simulink model "coolingskid_digitaltwin3"  (R2026a)
settings: Solver=VariableStepAuto  StopTime=10000
libraries: fl_lib x33, SimscapeFluids_lib x13, nesl_utility x12, slpidlib x1
settings Model: Creator=novik  LastModifiedBy=novik
settings SolverCC: MaxConsecutiveMinStep=2

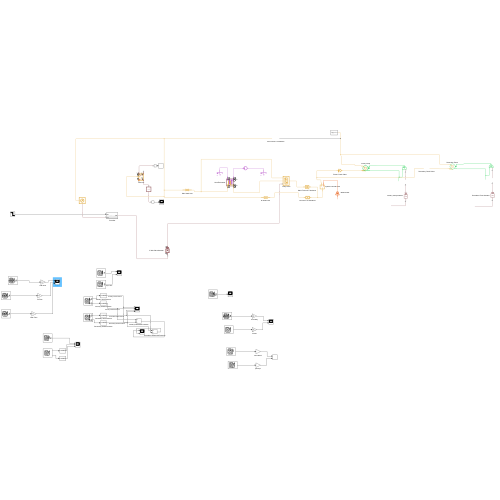
[thumbnail: Simulink's stored preview of the top-level diagram]
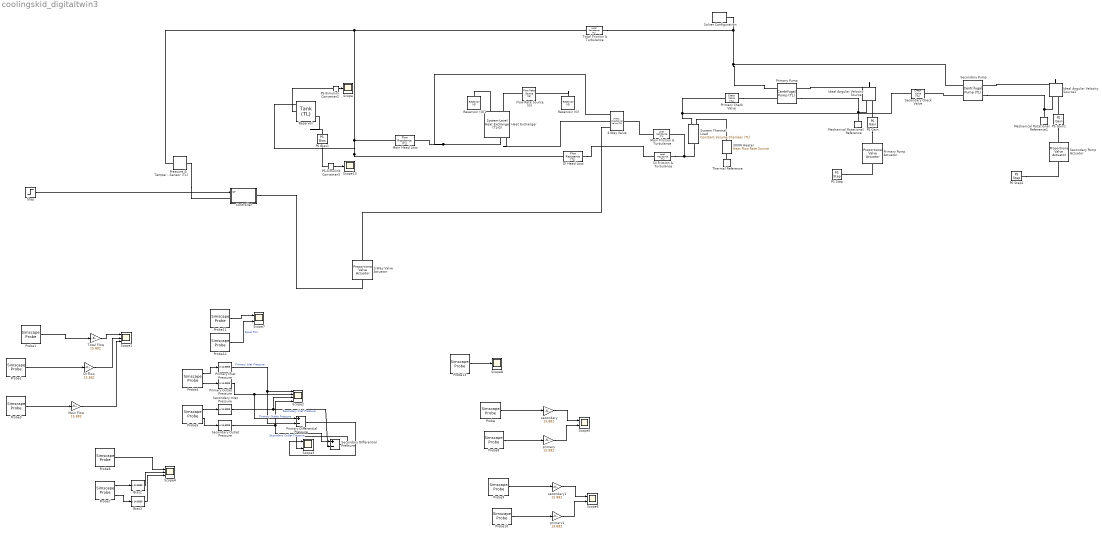
== system coolingskid_digitaltwin3 ==
  3-Way Valve : SimscapeFluids_lib/Thermal Liquid/Valves & Orifices/Directional Control Valves/3-Way Directional Valve (TL)  open_orifices_pos=fluids.thermal_liquid.valves.directional_control_valves.enum.OpenOrifices3Way.PA  open_orifices_neg=fluids.thermal_liquid.valves.directional_control_valves.enum.OpenOrifices3Way.AT  area_spec=fluids.thermal_liquid.valves.directional_control_valves.enum.area_spec.identical  valve_spec=fluids.thermal_liquid.valves.directional_control_valves.enum.ValveSpec.Linear  del_S_max=3e-3 m  area_max=0.502654824574 in^2  del_S_TLU=[0, .00125, .0025, .00375, .005] m  valve_area_TLU=[1e-10, 1e-05, 4e-05, 8e-05, .0001] m^2  del_S_flow_TLU=[0, .00125, .0025, .00375, .005] m  p_diff_TLU=[-.1, .3, .5, .7] MPa  vol_flow_TLU=[-9.05e-10, 1.57e-09, 2.02e-09, 2.39e-09; -9.05e-05, .000157, .000202, .000239; -.000362, .000627, .00081, .000958; -.000724, .00125, .00162, .00192; -.000905, .00156, .002, .00239] m^3/s  mdot_TLU=1e3 * [-9.05e-10, 1.57e-09, 2.02e-09, 2.39e-09; -9.05e-05, .000157, .000202, .000239; -.000362, .000627, .00081, .000958; -.000724, .00125, .00162, .00192; -.000905, .00156, .002, .00239] kg/s  T_ref_in=293.15 K  p_ref_in=0.101325 MPa  area_leak=1e-20 in^2  Cd=1  Re_c=1  smoothing_factor=0.01  pressure_recovery=false  area=0.533266503391 in^2  S_max_PA=5e-3 m  del_S_max_PA=0.005 m  area_max_PA=1e-4 m^2  del_S_TLU_PA=[0, .00125, .0025, .00375, .005] m  valve_area_TLU_PA=[1e-10, 1e-05, 4e-05, 8e-05, .0001] m^2  del_S_flow_TLU_PA=[0, .00125, .0025, .00375, .005] m  p_diff_TLU_PA=[-.1, .3, .5, .7] MPa  vol_flow_TLU_PA=[-9.05e-10, 1.57e-09, 2.02e-09, 2.39e-09; -9.05e-05, .000157, .000202, .000239; -.000362, .000627, .00081, .000958; -.000724, .00125, .00162, .00192; -.000905, .00156, .002, .00239] m^3/s  mdot_TLU_PA=1e3 * [-9.05e-10, 1.57e-09, 2.02e-09, 2.39e-09; -9.05e-05, .000157, .000202, .000239; -.000362, .000627, .00081, .000958; -.000724, .00125, .00162, .00192; -.000905, .00156, .002, .00239] kg/s  S_max_AT=0 m  del_S_max_AT=0.005 m  area_max_AT=1e-4 m^2  del_S_TLU_AT=[0, .00125, .0025, .00375, .005] m  valve_area_TLU_AT=[1e-10, 1e-05, 4e-05, 8e-05, .0001] m^2  del_S_flow_TLU_AT=[0, .00125, .0025, .00375, .005] m  p_diff_TLU_AT=[-.1, .3, .5, .7] MPa  vol_flow_TLU_AT=[-9.05e-10, 1.57e-09, 2.02e-09, 2.39e-09; -9.05e-05, .000157, .000202, .000239; -.000362, .000627, .00081, .000958; -.000724, .00125, .00162, .00192; -.000905, .00156, .002, .00239] m^3/s  mdot_TLU_AT=1e3 * [-9.05e-10, 1.57e-09, 2.02e-09, 2.39e-09; -9.05e-05, .000157, .000202, .000239; -.000362, .000627, .00081, .000958; -.000724, .00125, .00162, .00192; -.000905, .00156, .002, .00239] kg/s  S_max_PT=4.5e-3 m  del_S_max_PT=0.005 m  area_max_PT=1e-4 m^2  del_S_TLU_PT=[0, .00125, .0025, .00375, .005] m  valve_area_TLU_PT=[1e-10, 1e-05, 4e-05, 8e-05, .0001] m^2  del_S_flow_TLU_PT=[0, .00125, .0025, .00375, .005] m  p_diff_TLU_PT=[-.1, .3, .5, .7] MPa  vol_flow_TLU_PT=[-9.05e-10, 1.57e-09, 2.02e-09, 2.39e-09; -9.05e-05, .000157, .000202, .000239; -.000362, .000627, .00081, .000958; -.000724, .00125, .00162, .00192; -.000905, .00156, .002, .00239] m^3/s  mdot_TLU_PT=1e3 * [-9.05e-10, 1.57e-09, 2.02e-09, 2.39e-09; -9.05e-05, .000157, .000202, .000239; -.000362, .000627, .00081, .000958; -.000724, .00125, .00162, .00192; -.000905, .00156, .002, .00239] kg/s
  3-Way Valve Actuator : SimscapeFluids_lib/Valve Actuators/Proportional Valve Actuator  gain=5e-3 m  time_constant=3 s  valve_stroke=0.005 m
  300W Heater : fl_lib/Thermal/Thermal Sources/Heat Flow Rate Source  heat_flow=300 W
  Bias2 : Bias  Bias=-14.6959  SaturateOnIntegerOverflow=off
  Bias3 : Bias  Bias=-14.6959  SaturateOnIntegerOverflow=off
  Controller : Subsystem
  DI Flow : Gain  Gain=15.882
  DI Friction & Turbulance : SimscapeFluids_lib/Thermal Liquid/Pipes & Fittings/Local Resistance (TL)  resistance_loss_spec=fluids.thermal_liquid.pipes_fittings.enum.ResistanceLossSpec.Constant  loss_coeff_AB=0.041443  loss_coeff_BA=0.041443  Re_TLU=[-500, -200, -100, -50, -40, -30, -20, -10, 10, 20, 30, 40, 50, 100, 200, 500, 1000, 2000]  loss_coeff_TLU=[.65, .75, .9, 1.15, 1.35, 1.65, 2.3, 3.1, 4, 2.7, 1.8, 1.46, 1.3, .9, .65, .42, .3, .2]  flow_area=0.533266503391 in^2  Re_c=3380
  DI Head Loss : fl_lib/Thermal Liquid/Elements/Flow Resistance (TL)  delta_p_nominal=7.908 psi  mdot_nominal=0.05667 kg/s  area=0.533266503391 in^2  laminar_fraction=1e-3
  Flow Rate Source (G) : fl_lib/Gas/Sources/Flow Rate Source (G)  source_type=foundation.enum.constant_controlled.constant  flow_type=foundation.enum.mass_volumetric_flow.mass  mass_flow=5 kg/s  volumetric_flow=0 m^3/s  volumetric_flow_conditions=foundation.enum.volumetric_flow_conditions.standard  p_std=0.101325 MPa  T_std=20 degC  power_spec=foundation.enum.power_spec.isentropic  area_A=0.01 m^2  area_B=0.01 m^2
  Heat Exchanger : SimscapeFluids_lib/Heat Exchangers/Thermal Liquid - Gas/System-Level Heat Exchanger (TL-G)  flow_arrangement=fluids.heat_exchangers.enum.SystemLevelFlowArrangementTLG.Counter  wall_thermal_mass=false  mass_wall=1 kg  cp_wall=490 J/(K*kg)  nominal_init_wall=true  T_wall_init=293.15 K  area_A1=0.533266503391 in^2  area_B1=0.533266503391 in^2  area_A2=0.01 m^2  area_B2=0.01 m^2  operating_condition_TL=fluids.heat_exchangers.enum.SystemLevelOperatingConditionTLG.Cooling  mdot_nominal_TL=0.315450833333 kg/s  delta_p_nominal_TL=2.08 psi  p_in_nominal_TL=23.5 psi  T_in_nominal_TL=43.54 degC  capacity_spec_TL=fluids.heat_exchangers.enum.SystemLevelCapacitySpec.OutletCondition  Q_nominal=1 kW  T_out_nominal_TL=26.87 degC  volume_TL=.25 gal  nominal_init_TL=false  p_init_TL=1 atm  T_init_TL=25 degC  mdot_nominal_G=5 kg/s  delta_p_nominal_G=0.001 MPa  p_in_nominal_G=0.101325 MPa  T_in_nominal_G=25 degC  volume_G=0.1 m^3  nominal_init_G=true  p_init_G=0.101325 MPa  T_init_G=293.15 K  a_TL=0.023  b_TL=0.8  c_TL=0.33  a_G=0.023  b_G=0.8  c_G=0.33
  Ideal Angular Velocity Source : fl_lib/Mechanical/Mechanical Sources/Ideal Angular Velocity Source
  Ideal Angular Velocity Source1 : fl_lib/Mechanical/Mechanical Sources/Ideal Angular Velocity Source
  Main Flow : Gain  Gain=15.882
  Main Friction & Turbulance : SimscapeFluids_lib/Thermal Liquid/Pipes & Fittings/Local Resistance (TL)  resistance_loss_spec=fluids.thermal_liquid.pipes_fittings.enum.ResistanceLossSpec.Constant  loss_coeff_AB=0.026994  loss_coeff_BA=0.026994  Re_TLU=[-500, -200, -100, -50, -40, -30, -20, -10, 10, 20, 30, 40, 50, 100, 200, 500, 1000, 2000]  loss_coeff_TLU=[.65, .75, .9, 1.15, 1.35, 1.65, 2.3, 3.1, 4, 2.7, 1.8, 1.46, 1.3, .9, .65, .42, .3, .2]  flow_area=0.533266503391 in^2  Re_c=18778
  Main Head Loss : fl_lib/Thermal Liquid/Elements/Flow Resistance (TL)  delta_p_nominal=5.94 psi  mdot_nominal=0.315450833333 kg/s  area=0.533266503391 in^2  laminar_fraction=1e-3
  Mechanical Rotational Reference : fl_lib/Mechanical/Rotational Elements/Mechanical Rotational Reference
  Mechanical Rotational Reference1 : fl_lib/Mechanical/Rotational Elements/Mechanical Rotational Reference
  PS Bias1 : fl_lib/Physical Signals/Functions/PS Bias  bias=-273.15 K
  PS Gain : fl_lib/Physical Signals/Functions/PS Gain  gain=1 1/(m*s)
  PS Gain1 : fl_lib/Physical Signals/Functions/PS Gain  gain=1 1/(m*s)
  PS Step : fl_lib/Physical Signals/Sources/PS Step  step_time=5000 s  initial_value=1  final_value=0
  PS Step1 : fl_lib/Physical Signals/Sources/PS Step  step_time=5000 s  initial_value=0  final_value=1
  PS-Simulink Converter2 : nesl_utility/PS-Simulink Converter  PhysicalDomain=network_engine_domain  SubClassName=ps_output  LeftPortType=input  RightPortType=output  PseudoPeriodic=off  Frequencies=[]  VectorFormat=inherit  Unit=inherit  AffineConversion=off
  PS-Simulink Converter3 : nesl_utility/PS-Simulink Converter  PhysicalDomain=network_engine_domain  SubClassName=ps_output  LeftPortType=input  RightPortType=output  PseudoPeriodic=off  Frequencies=[]  VectorFormat=inherit  Unit=inherit  AffineConversion=off
  Pressure & Temperature Sensor (TL) : fl_lib/Thermal Liquid/Sensors/Pressure & Temperature Sensor (TL)  reference=foundation.enum.MeasurementReference.absolute  pressure=false  pressure_spec=foundation.enum.PressureMeasementSpec.Absolute  temperature=true
  Primary Check Valve : SimscapeFluids_lib/Thermal Liquid/Valves & Orifices/Directional Control Valves/Check Valve (TL)  opening_spec=fluids.thermal_liquid.valves.enum.PressureOpeningSpec.Linear  pressure_spec=fluids.thermal_liquid.valves.enum.PressureControlSpec.PressureDifferential  p_crack_gauge=0.1 MPa  p_crack_differential=0.01 psi  press_max_gauge=0.2 MPa  press_max_differential=0.21 psi  area_max=0.5 in^2  area_leak=1e-10 m^2  p_diff_TLU=[0.01 : 0.01 : 0.1] MPa  valve_area_TLU=[1e-10, 1e-05, 2e-05, 3e-05, 4e-05, 5e-05, 6e-05, 7.5e-05, 8.5e-05, .0001] m^2  vol_flow_TLU=[.000358, .045, .11, .191, .284, .39, .505, .63, .764, .905] .* 1e-3 m^3/s  area=0.533266503391 in^2  Cd=1  Re_c=1  smoothing_factor=0.01  pressure_recovery=false  opening_dynamics=false  tau=0.1 s
  Primary Differential Pressure : Sum  Inputs=+-
  Primary Inlet Pressure : Bias  Bias=-14.6959  SaturateOnIntegerOverflow=off
  Primary Outlet Pressure : Bias  Bias=-14.6959  SaturateOnIntegerOverflow=off
  Primary Pump : SimscapeFluids_lib/Thermal Liquid/Pumps & Motors/Centrifugal Pump (TL)  pump_parameterization=fluids.thermal_liquid.pumps_motors.enum.CentrifugalPumpParameterization.Nominal  capacity_ref_nominal=5.9 gpm  head_ref_nominal=19 ft  power_ref_nominal=0.02811289 kW  head_ref_max=20.7652445345097 ft  capacity_ref_max=31 gpm  omega_ref_analytic=1770 rpm  flow_rate_1D_TLU=[16.67, 30, 40, 53.33, 66.67, 83.33] lpm  head_1D_TLU=[50, 47.5, 45, 40, 35, 25] m  power_1D_TLU=[.6, .75, .85, .93, .98, .99] kW  omega_ref_1D=3500 rpm  rho_ref_1D=998.21 kg/m^3  omega_threshold_factor=1e-2  flow_rate_2D_TLU=[16.67, 23.33, 30, 40, 53.33, 60] lpm  omega_2D_TLU=[2450, 2800, 3150, 3500] rpm  head_2D_TLU=[25, 32.7, 42.5, 50; 24, 31.7, 41, 49; 22.7, 30.5, 39, 47.5; 20, 28, 36, 45; 15.7, 24, 32, 40; 12.5, 21, 29.5, 37.5] m  power_2D_TLU=[.28, .38, .5, .6; .31, .41, .55, .68; .33, .44, .6, .75; .36, .48, .65, .83; .38, .53, .72, .93; .39, .55, .75, .97] kW  rho_ref_2D=998.21 kg/m^3  diameter_ratio=1  mech_orientation=fluids.thermal_liquid.pumps_motors.enum.CentrifugalPumpMechOrientation.Positive  area=0.533266503391 in^2  operation_check=simscape.enum.assert.action.none
  Primary Pump Actuator : SimscapeFluids_lib/Valve Actuators/Proportional Valve Actuator  gain=185.3539665617978 m  time_constant=8 s  valve_stroke=185.3539665617978 m
  Probe : SimscapeProbe  BoundBlock=69  Variables="{\"mdot_A\":{\"Probing\":\"ON\"}}"
  Probe1 : SimscapeProbe  BoundBlock=421  Variables="{\"mdot_A\":{\"Probing\":\"ON\"}}"
  Probe10 : SimscapeProbe  BoundBlock=219  Variables="{\"O\":{\"Probing\":\"ON\"}}"
  Probe11 : SimscapeProbe  BoundBlock=406  Variables="{\"A.T\":{\"Unit\":\"degC\",\"Probing\":\"ON\"}}"
  Probe12 : SimscapeProbe  BoundBlock=118  Variables="{\"S\":{\"Probing\":\"ON\"}}"
  Probe13 : SimscapeProbe  BoundBlock=77  Variables="{\"B.p\":{\"Unit\":\"psi\",\"Probing\":\"ON\"}}"
  Probe2 : SimscapeProbe  BoundBlock=77  Variables="{\"mdot_A\":{\"Probing\":\"ON\"}}"
  Probe3 : SimscapeProbe  BoundBlock=73  Variables="{\"mdot_A\":{\"Probing\":\"ON\"}}"
  Probe4 : SimscapeProbe  BoundBlock=69  Variables="{\"A.p\":{\"Unit\":\"psi\",\"Probing\":\"ON\"},\"B.p\":{\"Unit\":\"psi\",\"Probing\":\"ON\"}}"
  Probe5 : SimscapeProbe  BoundBlock=236  Variables="{\"A.p\":{\"Unit\":\"psi\",\"Probing\":\"ON\"},\"B.p\":{\"Unit\":\"psi\",\"Probing\":\"ON\"},\"mdot_A\":{\"Probing\":\"OFF\"},\"mdot_B\":{\"Probing\":\"OFF\"}}"
  Probe6 : SimscapeProbe  BoundBlock=69  Variables="{\"R.w\":{\"Unit\":\"rpm\",\"Probing\":\"ON\"}}"
  Probe7 : SimscapeProbe  BoundBlock=69  Variables="{\"A.p\":{\"Unit\":\"psi\",\"Probing\":\"ON\"},\"B.p\":{\"Unit\":\"psi\",\"Probing\":\"ON\"}}"
  Probe8 : SimscapeProbe  BoundBlock=236  Variables="{\"mdot_A\":{\"Probing\":\"ON\"}}"
  Probe9 : SimscapeProbe  BoundBlock=240  Variables="{\"O\":{\"Probing\":\"ON\"}}"
  Reservoir : SimscapeFluids_lib/Thermal Liquid/Tanks & Accumulators/Tank (TL)  num_inlet=fluids.thermal_liquid.tanks_accumulators.enum.NumInlet.One  pressure_spec=fluids.thermal_liquid.tanks_accumulators.enum.TankPressureSpec.Atmospheric  tank_pressure=0.101325 MPa  volume_spec=fluids.thermal_liquid.tanks_accumulators.enum.TankVolumeSpec.Constant  tank_area=144 in^2  level_TLU=[0, 3, 5] m  volume_TLU=[0, 4, 6] m^3  inlet_height_A=0.1 in  inlet_area_A=.78 in^2  inlet_heights_AB=[.1, .1] m  inlet_areas_AB=[.01, .01] m^2  inlet_heights_ABC=[.1, .1, .1] m  inlet_areas_ABC=[.01, .01, .01] m^2  inlet_heights_ABCD=0.1 * ones(1, 4) m  inlet_areas_ABCD=0.01 * ones(1, 4) m^2  inlet_heights_ABCDE=0.1 * ones(1, 5) m  inlet_areas_ABCDE=0.01 * ones(1, 5) m^2  inlet_heights_ABCDEF=0.1 * ones(1, 6) m  inlet_areas_ABCDEF=0.01 * ones(1, 6) m^2  level_check=simscape.enum.assert.action.error  capacity_check=simscape.enum.assert.action.none  max_capacity=10 m^3  g=9.81 m/s^2  level_specify=on  level_priority=None  level=5 m  level_nominal_specify=off  level_nominal_value=1  level_nominal_unit=m  volume_specify=on  volume_priority=High  volume=4 gal  volume_nominal_specify=off  volume_nominal_value=4  volume_nominal_unit=gal  mass_specify=off  mass_priority=None  mass=5000 kg  mass_nominal_specify=off  mass_nominal_value=1  mass_nominal_unit=kg  T_I_specify=on  T_I_priority=High  T_I=25 degC  T_I_nominal_specify=off  T_I_nominal_value=1  T_I_nominal_unit=K
  Reservoir (G) : fl_lib/Gas/Elements/Reservoir (G)  pressure_input=false  pressure_spec=foundation.enum.pressure_spec.atmospheric  reservoir_pressure=0.101325 MPa  temperature_input=false  reservoir_temperature=25 degC  area_A=0.01 m^2  input_error_spec=foundation.enum.input_range_error.warn
  Reservoir (G)1 : fl_lib/Gas/Elements/Reservoir (G)  pressure_input=false  pressure_spec=foundation.enum.pressure_spec.atmospheric  reservoir_pressure=0.101325 MPa  temperature_input=false  reservoir_temperature=293.15 degC  area_A=0.01 m^2  input_error_spec=foundation.enum.input_range_error.warn
  Scope : Scope
      settings: ActiveDisplayYMinimum=0.01508889434891056  ActiveDisplayYMaximum=0.015292483650747727  DataLoggingVariableName=ScopeData5
  Scope1 : Scope  NumInputPorts=3
      settings: Title=Total Flow  ActiveDisplayYMinimum=6.1667689576391185  ActiveDisplayYMaximum=6.8690776559533306  YLabel=Flow (GPM)
  Scope13 : Scope
      settings: ActiveDisplayYMinimum=25.00428838938462  ActiveDisplayYMaximum=25.152201193488068  DataLoggingVariableName=ScopeData10
  Scope2 : Scope  NumInputPorts=4
      settings: ActiveDisplayYMinimum=-0.7997937937117674  ActiveDisplayYMaximum=9.44542911175904  YLabel=Pressure (psi)  DataLoggingVariableName=Pressure_Pump_PortA  DataLoggingSaveFormat=Array
  Scope{3,5..7} (4 alike) : Scope  NumInputPorts=2
      Scope3 settings: Title=Primary Differential Pressure  ActiveDisplayYMinimum=-1.0243925853144504  ActiveDisplayYMaximum=9.2217499271304018  YLabel=Pressure (psi)  DataLoggingVariableName=Pressure_Pump_PortA1  DataLoggingSaveFormat=Array
      Scope5 settings: ActiveDisplayYMinimum=1.077490568227446  ActiveDisplayYMaximum=7.5374604811752661  DataLoggingVariableName=ScopeData2
      Scope6 settings: ActiveDisplayYMinimum=-367.97396371923259  ActiveDisplayYMaximum=3311.7656592293288  DataLoggingVariableName=ScopeData3
      Scope7 settings: Title=Temperature  ActiveDisplayYMinimum=21.124726674032793  ActiveDisplayYMaximum=47.999112623350065  YLabel=Temp °C
  Scope4 : Scope  NumInputPorts=3
      settings: ActiveDisplayString=3  Title=Pump Outlet Pressure  ActiveDisplayYMinimum=-5.5996179237023327  ActiveDisplayYMaximum=310.42338582580572  YLabel=Pressure (psi)  DataLoggingVariableName=Pressure_Pump_PortA2  DataLoggingSaveFormat=Array
  Scope8 : Scope
      settings: ActiveDisplayYMinimum=14.00401391479239  ActiveDisplayYMaximum=15.025108344851473  YLabel=Flow (GPM)  DataLoggingVariableName=ScopeData4
  Secondary Check Valve : SimscapeFluids_lib/Thermal Liquid/Valves & Orifices/Directional Control Valves/Check Valve (TL)  opening_spec=fluids.thermal_liquid.valves.enum.PressureOpeningSpec.Linear  pressure_spec=fluids.thermal_liquid.valves.enum.PressureControlSpec.PressureDifferential  p_crack_gauge=0.1 MPa  p_crack_differential=0.01 psi  press_max_gauge=0.2 MPa  press_max_differential=0.21 psi  area_max=0.5 in^2  area_leak=1e-10 m^2  p_diff_TLU=[0.01 : 0.01 : 0.1] MPa  valve_area_TLU=[1e-10, 1e-05, 2e-05, 3e-05, 4e-05, 5e-05, 6e-05, 7.5e-05, 8.5e-05, .0001] m^2  vol_flow_TLU=[.000358, .045, .11, .191, .284, .39, .505, .63, .764, .905] .* 1e-3 m^3/s  area=0.533266503391 in^2  Cd=1  Re_c=1  smoothing_factor=0.01  pressure_recovery=false  opening_dynamics=false  tau=0.1 s
  Secondary Differential Pressure : Sum  Inputs=+-
  Secondary Inlet Pressure : Bias  Bias=-14.6959  SaturateOnIntegerOverflow=off
  Secondary Outlet Pressure : Bias  Bias=-14.6959  SaturateOnIntegerOverflow=off
  Secondary Pump : SimscapeFluids_lib/Thermal Liquid/Pumps & Motors/Centrifugal Pump (TL)  pump_parameterization=fluids.thermal_liquid.pumps_motors.enum.CentrifugalPumpParameterization.Nominal  capacity_ref_nominal=5.9 gpm  head_ref_nominal=19 ft  power_ref_nominal=0.02811289 kW  head_ref_max=20.7652445345097 ft  capacity_ref_max=31 gpm  omega_ref_analytic=1770 rpm  flow_rate_1D_TLU=[16.67, 30, 40, 53.33, 66.67, 83.33] lpm  head_1D_TLU=[50, 47.5, 45, 40, 35, 25] m  power_1D_TLU=[.6, .75, .85, .93, .98, .99] kW  omega_ref_1D=3500 rpm  rho_ref_1D=998.21 kg/m^3  omega_threshold_factor=1e-2  flow_rate_2D_TLU=[16.67, 23.33, 30, 40, 53.33, 60] lpm  omega_2D_TLU=[2450, 2800, 3150, 3500] rpm  head_2D_TLU=[25, 32.7, 42.5, 50; 24, 31.7, 41, 49; 22.7, 30.5, 39, 47.5; 20, 28, 36, 45; 15.7, 24, 32, 40; 12.5, 21, 29.5, 37.5] m  power_2D_TLU=[.28, .38, .5, .6; .31, .41, .55, .68; .33, .44, .6, .75; .36, .48, .65, .83; .38, .53, .72, .93; .39, .55, .75, .97] kW  rho_ref_2D=998.21 kg/m^3  diameter_ratio=1  mech_orientation=fluids.thermal_liquid.pumps_motors.enum.CentrifugalPumpMechOrientation.Positive  area=0.533266503391 in^2  operation_check=simscape.enum.assert.action.none
  Secondary Pump Actuator : SimscapeFluids_lib/Valve Actuators/Proportional Valve Actuator  gain=185.3539665617978 m  time_constant=8 s  valve_stroke=185.3539665617978 m
  Solver Configuration : nesl_utility/Solver Configuration  PhysicalDomain=network_engine_domain  SubClassName=solver  LeftPortType=input  RightPortType=generic  Tones=[]  Harmonics=[]  SimulateNoise=off  Profile=off  UseLocalSampling=off  EnableSwitchedLinearOptims=on  FrequencyDomain=off  UseCCode=off  RelTol=0.001  AbsTol=0.001  MinStep=1e-09  ToWorkspace=off  RevertToSquareIcSolve=off  NumHomotopyIterations=100  PhasorMode=off  PhasorModeNumHarmonics=1  ConsistencySolver=NEWTON_XTOL_AFTER_FTOL  CanonicalOrdering=CANONICAL  OptimizeIntermediates=OPTIMIZED  IndexReductionMethod=DerivativeReplacement  DoDC=off  ResidualTolerance=1e-09  ConsistencyTolSource=GLOBAL  ConsistencyAbsTol=0.001  ConsistencyRelTol=0.001  ConsistencyTolFactor=0.001  UseLocalSolver=off  LocalSolverChoice=NE_TRAPEZOIDAL_ADVANCER  ResolveIndetEquations=on  FunctionEvalNumThread=1  LocalSolverSampleTime=0.001  DoFixedCost=off  MaxNonlinIter=3  MaxModeIter=2  ComputeImpulses=off  ImpulseIterations=2  LinearAlgebra=auto  LinearAlgebraNumThread=0  EquationFormulation=NE_TIME_EF  DelaysMemoryBudget=1024  AutomaticFiltering=on  FilteringTimeConstant=0.001  PartitionStorageMethod=AS_NEEDED  PartitionMemoryBudget=1024  PartitionMethod=FAST  MultibodyUseLocalSolver=off  MultibodyLocalSolverChoice=ODE1  MultibodyLocalSolverSampleTime=0.001
  Step : Step  Time=6000  InitialValue=45  FinalValue=37  SampleTime=0
  System Thermal Load : fl_lib/Thermal Liquid/Elements/Constant Volume Chamber (TL)  volume=4.38 gal  num_ports=foundation.enum.num_ports.two  area_A=0.533266503391 in^2  area_B=0.533266503391 in^2  area_C=0.01 m^2  area_D=0.01 m^2  p_I_specify=off  p_I_priority=High  p_I=0.101325 MPa  p_I_nominal_specify=off  p_I_nominal_value=1  p_I_nominal_unit=MPa  T_I_specify=off  T_I_priority=High  T_I=293.15 K  T_I_nominal_specify=off  T_I_nominal_value=1  T_I_nominal_unit=K  u_I_specify=off  u_I_priority=None  u_I=83.906 kJ/kg  u_I_nominal_specify=off  u_I_nominal_value=1  u_I_nominal_unit=kJ/kg  rho_I_specify=off  rho_I_priority=None  rho_I=998.21 kg/m^3  rho_I_nominal_specify=off  rho_I_nominal_value=1  rho_I_nominal_unit=kg/m^3
  Thermal Reference : fl_lib/Thermal/Thermal Elements/Thermal Reference
  "Total Flow " : Gain  Gain=15.882
  Total Friction & Turbulance : SimscapeFluids_lib/Thermal Liquid/Pipes & Fittings/Local Resistance (TL)  resistance_loss_spec=fluids.thermal_liquid.pipes_fittings.enum.ResistanceLossSpec.Constant  loss_coeff_AB=0.025900  loss_coeff_BA=0.025900  Re_TLU=[-500, -200, -100, -50, -40, -30, -20, -10, 10, 20, 30, 40, 50, 100, 200, 500, 1000, 2000]  loss_coeff_TLU=[.65, .75, .9, 1.15, 1.35, 1.65, 2.3, 3.1, 4, 2.7, 1.8, 1.46, 1.3, .9, .65, .42, .3, .2]  flow_area=0.533266503391 in^2  Re_c=22159
  primary : Gain  Gain=15.882
  primary1 : Gain  Gain=15.882
  secondary : Gain  Gain=15.882
  secondary1 : Gain  Gain=15.882
  wires:
  "Total Flow "/1 -> Scope1/1
  Probe2/1 -> DI Flow/1
  DI Flow/1 -> Scope1/2
  Probe3/1 -> Main Flow/1
  Main Flow/1 -> Scope1/3
  Probe5/1 -> Secondary Inlet Pressure/1
  Secondary Inlet Pressure/1 -> Secondary Differential Pressure/2, Scope2/3  "Secondary Inlet Pressure"
  Probe5/2 -> Secondary Outlet Pressure/1
  Secondary Outlet Pressure/1 -> Secondary Differential Pressure/1, Scope2/4  "Secondary Outlet Pressure"
  Secondary Differential Pressure/1 -> Scope3/2
  Probe7/1 -> Bias2/1
  Bias2/1 -> Scope4/2
  Bias3/1 -> Scope4/3
  Probe7/2 -> Bias3/1
  Probe6/1 -> Scope4/1
  Probe/1 -> secondary/1
  Probe8/1 -> primary/1
  secondary/1 -> Scope5/1
  primary/1 -> Scope5/2
  Probe10/1 -> primary1/1
  secondary1/1 -> Scope6/1
  primary1/1 -> Scope6/2
  Probe9/1 -> secondary1/1
  Probe4/1 -> Primary Inlet Pressure/1
  Probe4/2 -> Primary Outlet Pressure/1
  Primary Outlet Pressure/1 -> Primary Differential Pressure/1, Scope2/2  "Primary Outlet Pressure"
  Primary Inlet Pressure/1 -> Primary Differential Pressure/2, Scope2/1  "Primary Inlet Pressure"
  Primary Differential Pressure/1 -> Scope3/1
  Probe12/1 -> Scope7/2  "Spool Pos"
  PS-Simulink Converter2/1 -> Scope/1
  Probe11/1 -> Scope7/1
  Probe1/1 -> "Total Flow "/1
  PS-Simulink Converter3/1 -> Scope13/1
  Step/1 -> Controller/1(SP)
  Probe13/1 -> Scope8/1
  connections:
  Primary Pump/RConn2 -- Mechanical Rotational Reference/LConn1 -- Ideal Angular Velocity Source/RConn2
  Reservoir (G)/LConn1 -- Flow Rate Source (G)/LConn1
  Flow Rate Source (G)/RConn1 -- Heat Exchanger/RConn1
  Heat Exchanger/RConn2 -- Reservoir (G)1/LConn1
  Heat Exchanger/LConn2 -- 3-Way Valve/RConn3 -- Main Head Loss/LConn1
  DI Head Loss/LConn1 -- DI Friction & Turbulance/LConn1
  Main Friction & Turbulance/LConn1 -- 3-Way Valve/LConn1
  3-Way Valve/RConn2 -- Heat Exchanger/LConn1
  DI Friction & Turbulance/RConn1 -- System Thermal Load/RConn1 -- Main Friction & Turbulance/RConn1
  Ideal Angular Velocity Source/LConn1 -- Primary Pump/RConn1
  PS Step/RConn1 -- Primary Pump Actuator/LConn1
  PS Gain/RConn1 -- Ideal Angular Velocity Source/RConn1
  PS Gain/LConn1 -- Primary Pump Actuator/RConn1
  Solver Configuration/RConn1 -- Total Friction & Turbulance/RConn1 -- Secondary Pump/LConn1 -- Primary Pump/LConn1
  Primary Check Valve/LConn1 -- Primary Pump/LConn2
  Ideal Angular Velocity Source1/RConn2 -- Mechanical Rotational Reference1/LConn1 -- Secondary Pump/RConn2
  Secondary Pump/LConn2 -- Secondary Check Valve/LConn1
  PS Step1/RConn1 -- Secondary Pump Actuator/LConn1
  Ideal Angular Velocity Source1/LConn1 -- Secondary Pump/RConn1
  PS Gain1/RConn1 -- Ideal Angular Velocity Source1/RConn1
  PS Gain1/LConn1 -- Secondary Pump Actuator/RConn1
  PS-Simulink Converter2/LConn1 -- Reservoir/LConn2
  Main Head Loss/RConn1 -- Pressure & Temperature Sensor (TL)/LConn1 -- Total Friction & Turbulance/LConn1 -- Reservoir/LConn1 -- DI Head Loss/RConn1
  Primary Check Valve/RConn1 -- System Thermal Load/LConn1 -- Secondary Check Valve/RConn1
  Thermal Reference/LConn1 -- 300W Heater/RConn1
  300W Heater/LConn1 -- System Thermal Load/LConn2
  PS Bias1/LConn1 -- Reservoir/RConn2
  PS Bias1/RConn1 -- PS-Simulink Converter3/LConn1
  Pressure & Temperature Sensor (TL)/RConn1 -- Controller/LConn1
  3-Way Valve Actuator/RConn1 -- 3-Way Valve/RConn1
  Controller/RConn1 -- 3-Way Valve Actuator/LConn1

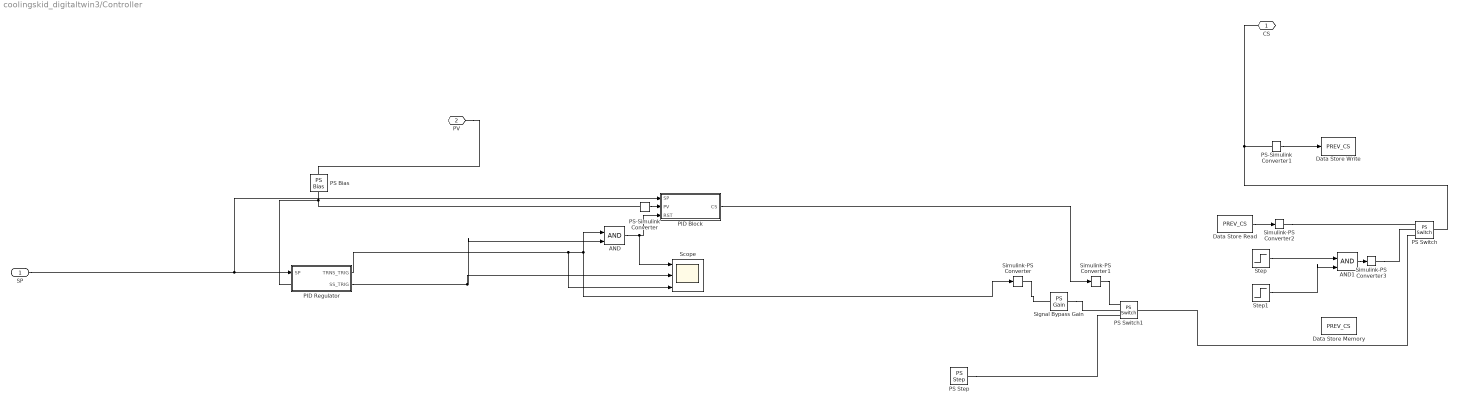
== system coolingskid_digitaltwin3/Controller ==
  SP : Inport
  AND : Logic  IconShape=distinctive  AllPortsSameDT=off  OutDataTypeStr=boolean
  AND1 : Logic  IconShape=distinctive  AllPortsSameDT=off  OutDataTypeStr=Inherit: Inherit via back propagation
  Data Store Memory : DataStoreMemory  DataStoreName=PREV_CS  WriteAfterWriteMsg=warning  ShowAdditionalParam=off
  Data Store Read : DataStoreRead  DataStoreName=PREV_CS  IndexOptions=Index vector (dialog)  Indices=1  OutputSizes=1
  Data Store Write : DataStoreWrite  DataStoreName=PREV_CS  IndexOptions=Index vector (dialog)  Indices=1  OutputSizes=1
  PID Block : Subsystem
  PID Regulator : Subsystem
  PS Bias : fl_lib/Physical Signals/Functions/PS Bias  bias=-273.15 K
  PS Step : fl_lib/Physical Signals/Sources/PS Step  step_time=250 s  initial_value=1  final_value=0
  PS Switch : fl_lib/Physical Signals/Nonlinear Operators/PS Switch  Threshold=0.5  ZeroCross=true
  PS Switch1 : fl_lib/Physical Signals/Nonlinear Operators/PS Switch  Threshold=0.5  ZeroCross=true
  PS-Simulink Converter : nesl_utility/PS-Simulink Converter  PhysicalDomain=network_engine_domain  SubClassName=ps_output  LeftPortType=input  RightPortType=output  PseudoPeriodic=off  Frequencies=[]  VectorFormat=inherit  Unit=inherit  AffineConversion=off
  PS-Simulink Converter1 : nesl_utility/PS-Simulink Converter  PhysicalDomain=network_engine_domain  SubClassName=ps_output  LeftPortType=input  RightPortType=output  PseudoPeriodic=off  Frequencies=[]  VectorFormat=inherit  Unit=inherit  AffineConversion=off
  Scope : Scope  NumInputPorts=3
      settings: ActiveDisplayYMinimum=-0.12228218018428028  ActiveDisplayYMaximum=1.1902178198157203  DataLoggingVariableName=ScopeData7
  Signal Bypass Gain : fl_lib/Physical Signals/Functions/PS Gain  gain=1
  Simulink-PS Converter{,1..3} (4 alike) : nesl_utility/Simulink-PS Converter  PhysicalDomain=network_engine_domain  SubClassName=ps_input  LeftPortType=input  RightPortType=output  PseudoPeriodic=off  Frequencies=[]  NoiseDistribution=none  NoiseParameters=[]  Unit=1  AffineConversion=off  FilteringAndDerivatives=provide  SimscapeFilterOrder=1  InputFilterTimeConstant=0.001  UdotUserProvided=0
  Step : Step  Time=5000  OutDataTypeStr=Inherit: Inherit via back propagation  SampleTime=0
  Step1 : Step  Time=5020  InitialValue=1  FinalValue=0  OutDataTypeStr=Inherit: Inherit via back propagation  SampleTime=0
  CS : PMIOPort  Side=Right
  PV : PMIOPort  Port=2  Side=Left
  wires:
  PID Block/1(CS) -> Simulink-PS Converter1/1
  SP/1 -> PID Regulator/1(SP), PID Block/1(SP)
  AND/1 -> Scope/1, PID Block/3(RST)
  PID Regulator/1(TRNS_TRIG) -> Scope/3, Simulink-PS Converter/1, AND/1
  PID Regulator/2(SS_TRIG) -> Scope/2, AND/2
  PS-Simulink Converter/1 -> PID Block/2(PV)
  PS-Simulink Converter1/1 -> Data Store Write/1
  Data Store Read/1 -> Simulink-PS Converter2/1
  Step/1 -> AND1/1
  Step1/1 -> AND1/2
  AND1/1 -> Simulink-PS Converter3/1
  connections:
  PS Bias/RConn1 -- PS-Simulink Converter/LConn1 -- PID Regulator/LConn1
  PS Switch/LConn3 -- PS Switch1/RConn1
  Simulink-PS Converter1/RConn1 -- PS Switch1/LConn1
  Simulink-PS Converter/RConn1 -- Signal Bypass Gain/LConn1
  PV/RConn1 -- PS Bias/LConn1
  Signal Bypass Gain/RConn1 -- PS Switch1/LConn2
  PS Step/RConn1 -- PS Switch1/LConn3
  Simulink-PS Converter2/RConn1 -- PS Switch/LConn1
  Simulink-PS Converter3/RConn1 -- PS Switch/LConn2
  CS/RConn1 -- PS Switch/RConn1 -- PS-Simulink Converter1/LConn1

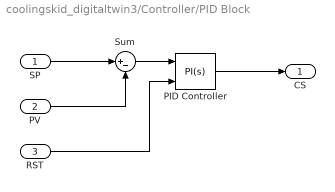
== system coolingskid_digitaltwin3/Controller/PID Block ==
  SP : Inport
  PV : Inport  Port=2
  RST : Inport  Port=3
  PID Controller : slpidlib/PID Controller  Controller=PI  Form=Parallel  TimeDomain=Continuous-time  UseExternalTs=off  SampleTime=-1  IntegratorMethod=Forward Euler  FilterMethod=Forward Euler  ControllerParametersSource=internal  P=-0.4  I=-0.03  UseKiTs=off  D=-0.3  UseExternalDerivativeSource=off  N=100  UseFilter=on  TunerSelectOption=Transfer Function Based (PID Tuner App)  InitialConditionSource=internal  InitialConditionForIntegrator=0  InitialConditionForFilter=0  DifferentiatorICPrevScaledInput=0  ExternalReset=rising  TrackingMode=off  Kt=1  LimitOutput=off  SatLimitsSource=internal  UpperSaturationLimit=inf  LowerSaturationLimit=-inf  LinearizeAsGain=on  AntiWindupMode=none  Kb=1  LimitIntegrator=off  UpperIntegratorSaturationLimit=inf  LowerIntegratorSaturationLimit=-inf  POutMin=[]  POutMax=[]  IOutMin=[]  IOutMax=[]  DOutMin=[]  DOutMax=[]  NOutMin=[]  NOutMax=[]  SumOutMin=[]  SumOutMax=[]  SaturationOutMin=[]  SaturationOutMax=[]  PParamMin=[]  PParamMax=[]  IParamMin=[]  IParamMax=[]  DParamMin=[]  DParamMax=[]  NParamMin=[]  NParamMax=[]  KbParamMin=[]  KbParamMax=[]  KtParamMin=[]  KtParamMax=[]  KbOutMin=[]  KbOutMax=[]  KtOutMin=[]  KtOutMax=[]  IntegratorOutMin=[]  IntegratorOutMax=[]  FilterOutMin=[]  FilterOutMax=[]  SumI1OutMin=[]  SumI1OutMax=[]  SumI2OutMin=[]  SumI2OutMax=[]  SumI3OutMin=[]  SumI3OutMax=[]  SumI4OutMin=[]  SumI4OutMax=[]  SumDOutMin=[]  SumDOutMax=[]  DifferentiatorOutMin=[]  DifferentiatorOutMax=[]  FilterDiffOutCoefMin=[]  FilterDiffOutCoefMax=[]  ReciprocalOutMin=[]  ReciprocalOutMax=[]  SumDenOutMin=[]  SumDenOutMax=[]  SumNumOutMin=[]  SumNumOutMax=[]  DivideOutMin=[]  DivideOutMax=[]  UdiffTsProdOutMin=[]  UdiffTsProdOutMax=[]  NTsProdOutMin=[]  NTsProdOutMax=[]  UintegralTsProdOutMin=[]  UintegralTsProdOutMax=[]  UngainTsProdOutMin=[]  UngainTsProdOutMax=[]  ClampingZeroOutDataTypeStr=Inherit: Inherit via back propagation  ClampingZeroOutMin=[]  ClampingZeroOutMax=[]  FilterDenConstantOutDataTypeStr=Inherit: Inherit via back propagation  FilterDenConstantOutMin=[]  FilterDenConstantOutMax=[]  PCopyOutDataTypeStr=Inherit: Inherit via back propagation  PCopyOutMin=[]  PCopyOutMax=[]  NCopyOutDataTypeStr=Inherit: Inherit via back propagation  NCopyOutMin=[]  NCopyOutMax=[]  IntegratorContinuousStateAttributes=''  IntegratorStateMustResolveToSignalObject=off  IntegratorRTWStateStorageClass=Auto  FilterContinuousStateAttributes=''  FilterStateMustResolveToSignalObject=off  FilterRTWStateStorageClass=Auto  ParallelPVariant=InternalParameters  IdealPVariant=Disabled  IVariant=InternalParameters  DVariant=Disabled  IntegratorVariant=Continuous  SatVariant=Disabled  AWVariant=Passthrough  PCopyVariant=Disabled  TRVariant=Disabled  FdbkBlocksVariant=Forward  IdealPFdbkVariant=Disabled  SatFdbkVariant=Disabled  DerivativeFilterVariant=Disabled  NVariant=Disabled  NCopyVariant=Disabled_SignalSpec  FilterICVariant=Disabled  IntegratorICVariant=InternalICs  ExternalResetVariant=ExternalReset  TRSumVariant=Passthrough  SumFdbkVariant=Disabled  SumVariant=Sum_PI  TsampFilterVariant=InternalTs  TsampNgainVariant=Passthrough  TsampIntegralVariant=Disabled_SignalSpec  ExternalSaturationOutDataTypeStr=Inherit: Same as second input  DerivativeSourceVariant=Disabled  PreIntVariant=InternalPreInt
  Sum : Sum  Inputs=|+-
  CS : Outport
  wires:
  RST/1 -> PID Controller/2
  SP/1 -> Sum/1
  PV/1 -> Sum/2
  PID Controller/1 -> CS/1
  Sum/1 -> PID Controller/1

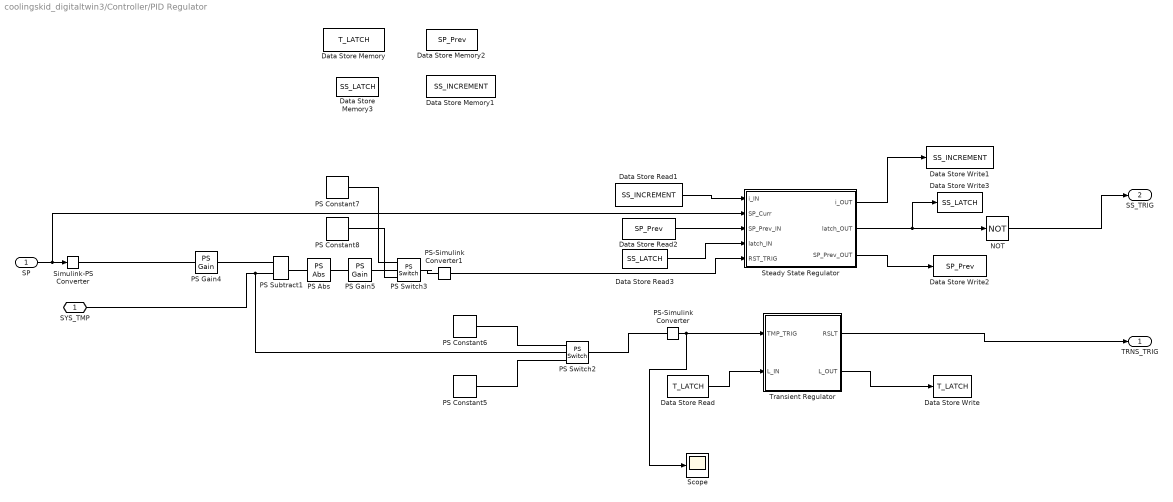
== system coolingskid_digitaltwin3/Controller/PID Regulator ==
  SP : Inport
  Data Store Memory : DataStoreMemory  DataStoreName=T_LATCH  WriteAfterWriteMsg=warning  ShowAdditionalParam=off
  Data Store Memory1 : DataStoreMemory  DataStoreName=SS_INCREMENT  WriteAfterWriteMsg=warning  ShowAdditionalParam=off
  Data Store Memory2 : DataStoreMemory  DataStoreName=SP_Prev  WriteAfterWriteMsg=warning  ShowAdditionalParam=off
  Data Store Memory3 : DataStoreMemory  DataStoreName=SS_LATCH  WriteAfterWriteMsg=warning  ShowAdditionalParam=off
  Data Store Read : DataStoreRead  DataStoreName=T_LATCH  IndexOptions=Index vector (dialog)  Indices=1  OutputSizes=1
  Data Store Read1 : DataStoreRead  DataStoreName=SS_INCREMENT  IndexOptions=Index vector (dialog)  Indices=1  OutputSizes=1
  Data Store Read2 : DataStoreRead  DataStoreName=SP_Prev  IndexOptions=Index vector (dialog)  Indices=1  OutputSizes=1
  Data Store Read3 : DataStoreRead  DataStoreName=SS_LATCH  IndexOptions=Index vector (dialog)  Indices=1  OutputSizes=1
  Data Store Write : DataStoreWrite  DataStoreName=T_LATCH  IndexOptions=Index vector (dialog)  Indices=1  OutputSizes=1
  Data Store Write1 : DataStoreWrite  DataStoreName=SS_INCREMENT  IndexOptions=Index vector (dialog)  Indices=1  OutputSizes=1
  Data Store Write2 : DataStoreWrite  DataStoreName=SP_Prev  IndexOptions=Index vector (dialog)  Indices=1  OutputSizes=1
  Data Store Write3 : DataStoreWrite  DataStoreName=SS_LATCH  IndexOptions=Index vector (dialog)  Indices=1  OutputSizes=1
  NOT : Logic  Operator=NOT  IconShape=distinctive  AllPortsSameDT=off  OutDataTypeStr=boolean
  PS Abs : fl_lib/Physical Signals/Nonlinear Operators/PS Abs  ZeroCross=true
  PS Constant5 : fl_lib/Physical Signals/Sources/PS Constant  constant=0
  PS Constant6 : fl_lib/Physical Signals/Sources/PS Constant  constant=1
  PS Constant7 : fl_lib/Physical Signals/Sources/PS Constant  constant=1
  PS Constant8 : fl_lib/Physical Signals/Sources/PS Constant  constant=0
  PS Gain4 : fl_lib/Physical Signals/Functions/PS Gain  gain=1 K
  PS Gain5 : fl_lib/Physical Signals/Functions/PS Gain  gain=-1
  PS Subtract1 : fl_lib/Physical Signals/Functions/PS Subtract
  PS Switch2 : fl_lib/Physical Signals/Nonlinear Operators/PS Switch  Threshold=45 K  ZeroCross=true
  PS Switch3 : fl_lib/Physical Signals/Nonlinear Operators/PS Switch  Threshold=-1 K  ZeroCross=true
  PS-Simulink Converter : nesl_utility/PS-Simulink Converter  PhysicalDomain=network_engine_domain  SubClassName=ps_output  LeftPortType=input  RightPortType=output  PseudoPeriodic=off  Frequencies=[]  VectorFormat=inherit  Unit=inherit  AffineConversion=off
  PS-Simulink Converter1 : nesl_utility/PS-Simulink Converter  PhysicalDomain=network_engine_domain  SubClassName=ps_output  LeftPortType=input  RightPortType=output  PseudoPeriodic=off  Frequencies=[]  VectorFormat=inherit  Unit=inherit  AffineConversion=off
  Scope : Scope
      settings: ActiveDisplayYMinimum=-1  ActiveDisplayYMaximum=1  DataLoggingVariableName=ScopeData6
  Simulink-PS Converter : nesl_utility/Simulink-PS Converter  PhysicalDomain=network_engine_domain  SubClassName=ps_input  LeftPortType=input  RightPortType=output  PseudoPeriodic=off  Frequencies=[]  NoiseDistribution=none  NoiseParameters=[]  Unit=1  AffineConversion=off  FilteringAndDerivatives=provide  SimscapeFilterOrder=1  InputFilterTimeConstant=0.001  UdotUserProvided=0
  Steady State Regulator : MATLAB Function  TreatAsAtomicUnit=on
  Transient Regulator : MATLAB Function  TreatAsAtomicUnit=on
  SYS_TMP : PMIOPort  Side=Left
  TRNS_TRIG : Outport
  SS_TRIG : Outport  Port=2
  wires:
  Data Store Read/1 -> Transient Regulator/2(L_IN)
  Transient Regulator/2(L_OUT) -> Data Store Write/1
  PS-Simulink Converter/1 -> Scope/1, Transient Regulator/1(TMP_TRIG)
  Transient Regulator/1(RSLT) -> TRNS_TRIG/1
  PS-Simulink Converter1/1 -> Steady State Regulator/5(RST_TRIG)
  SP/1 -> Steady State Regulator/2(SP_Curr), Simulink-PS Converter/1
  Data Store Read2/1 -> Steady State Regulator/3(SP_Prev_IN)
  Steady State Regulator/3(SP_Prev_OUT) -> Data Store Write2/1
  Data Store Read3/1 -> Steady State Regulator/4(latch_IN)
  Steady State Regulator/2(latch_OUT) -> Data Store Write3/1, NOT/1
  Data Store Read1/1 -> Steady State Regulator/1(i_IN)
  Steady State Regulator/1(i_OUT) -> Data Store Write1/1
  NOT/1 -> SS_TRIG/1
  connections:
  PS Subtract1/LConn2 -- PS Switch2/LConn2 -- SYS_TMP/RConn1
  Simulink-PS Converter/RConn1 -- PS Gain4/LConn1
  PS Constant7/RConn1 -- PS Switch3/LConn1
  PS Constant8/RConn1 -- PS Switch3/LConn3
  PS Abs/LConn1 -- PS Subtract1/RConn1
  PS-Simulink Converter/LConn1 -- PS Switch2/RConn1
  PS Gain5/LConn1 -- PS Abs/RConn1
  PS Switch3/LConn2 -- PS Gain5/RConn1
  PS Constant6/RConn1 -- PS Switch2/LConn1
  PS Subtract1/LConn1 -- PS Gain4/RConn1
  PS Constant5/RConn1 -- PS Switch2/LConn3
  PS Switch3/RConn1 -- PS-Simulink Converter1/LConn1

== matlab function coolingskid_digitaltwin3/Controller/PID Regulator/Transient Regulator ==
  data: RSLT output; TMP_TRIG input; L_IN input; L_OUT output
function [RSLT, L_OUT] = PID_Trans_Regulator(TMP_TRIG, L_IN)
    if TMP_TRIG == 1 && L_IN == 0
        RSLT = 1;
        L_OUT = 1;
    elseif TMP_TRIG == 1 && L_IN == 1
        RSLT = 1;
        L_OUT = 1;
    elseif TMP_TRIG == 0 && L_IN == 1
        RSLT = 1;
        L_OUT = 1;
    elseif TMP_TRIG == 0 && L_IN == 0
        RSLT = 0;
        L_OUT = 0;
    else
        RSLT = 0;
        L_OUT = 0;
    end

== matlab function coolingskid_digitaltwin3/Controller/PID Regulator/Steady State Regulator ==
  data: i_IN input; i_OUT output; SP_Curr input; latch_OUT output; SP_Prev_IN input; latch_IN input; RST_TRIG input; SP_Prev_OUT output
function [i_OUT, latch_OUT, SP_Prev_OUT] = PID_SS_Regulator(i_IN, SP_Curr, SP_Prev_IN, latch_IN, RST_TRIG)
if (i_IN > 0)
if (latch_IN == 1)
    if(RST_TRIG == 1)
        SP_Prev_OUT = SP_Curr;
        latch_OUT = 0;
    else
        SP_Prev_OUT = SP_Prev_IN;
        latch_OUT = 1;
    end
else
    if (SP_Prev_IN ~= SP_Curr)
        SP_Prev_OUT = SP_Prev_IN;
        latch_OUT = 1;
    else
        SP_Prev_OUT = SP_Curr;
        latch_OUT = 0;
    end
end
i_OUT = 1;
else
    i_OUT = 1;
    SP_Prev_OUT = SP_Curr;
    latch_OUT = 0;
end
